simulink model "weld_monitor"  (R2025b)
settings: Solver=FixedStepDiscrete  StartTime=0.0  StopTime=2  FixedStep=0.0001  RelTol=1e-3
values from neighbouring files (symbols this model uses):
  TH_burn_rms = thresholds_struct.burn_rms    [weld_simulink_prep.m]    (also in weld_simulink_workspace.mat = 2.1607081374)
libraries: dspstat3 x1
settings Model: Creator=pkhan  LastModifiedBy=pkhan

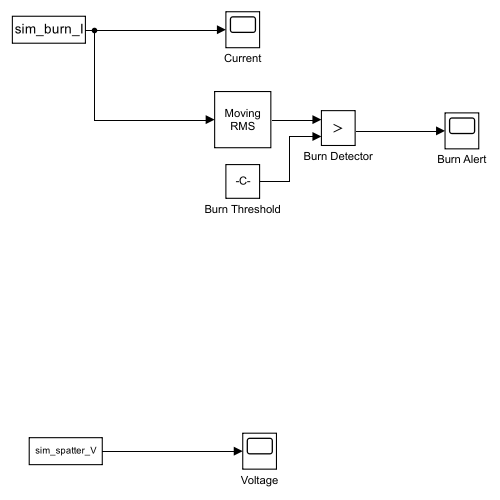
[thumbnail: Simulink's stored preview of the top-level diagram]
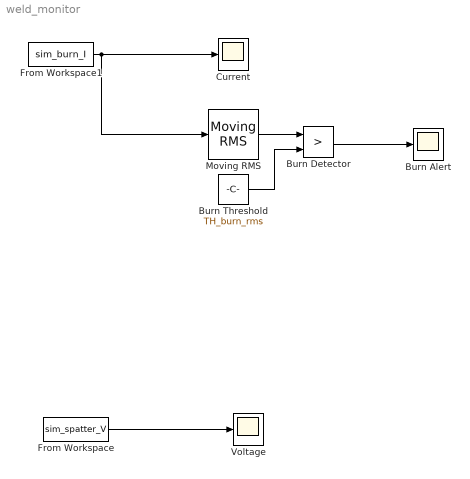
== system weld_monitor ==
  Burn Alert : Scope
      settings: ActiveDisplayYMinimum=-15.007239097379944  ActiveDisplayYMaximum=12.900173945290977  DataLoggingVariableName=ScopeData2
  Burn Detector : RelationalOperator  Operator=>  OutDataTypeStr=boolean  RndMeth=Simplest  InputSameDT=off
  Burn Threshold : Constant  Value=TH_burn_rms
  Current : Scope
      settings: ActiveDisplayYMinimum=1.2901676522777052  ActiveDisplayYMaximum=2.2678019071640181
  From Workspace : FromWorkspace  VariableName=sim_spatter_V  SampleTime=0.0001
  From Workspace1 : FromWorkspace  VariableName=sim_burn_I  SampleTime=0.0001
  Moving RMS : dspstat3/Moving RMS  Method=Sliding window  ForgettingFactorPort=off  SpecifyWindowLength=on  WindowLength=1000  OverlapLength=0  AllowArbitraryInputLength=on  ForgettingFactor=0.9  SimulateUsing=Interpreted execution
  Voltage : Scope
      settings: ActiveDisplayYMinimum=-1  ActiveDisplayYMaximum=1
  wires:
  From Workspace/1 -> Voltage/1
  From Workspace1/1 -> Moving RMS/1, Current/1
  Moving RMS/1 -> Burn Detector/1
  Burn Threshold/1 -> Burn Detector/2
  Burn Detector/1 -> Burn Alert/1
